simulink model "SrmAmLinearApcZhw3b1"  (R2013b)
settings: Solver=ode45  StartTime=0.0  StopTime=0.1  RelTol=1e-3
InitFcn:
  | theta0=30*2*pi/360;
  | ks=1.22;
  | is=2;
  | lu=0.016;
  | rs=1.5;
  | lux=1;
  | j=0.005;
settings Model: NumberOfSteps=5  Creator=mamingkai  LastModifiedBy=Think79

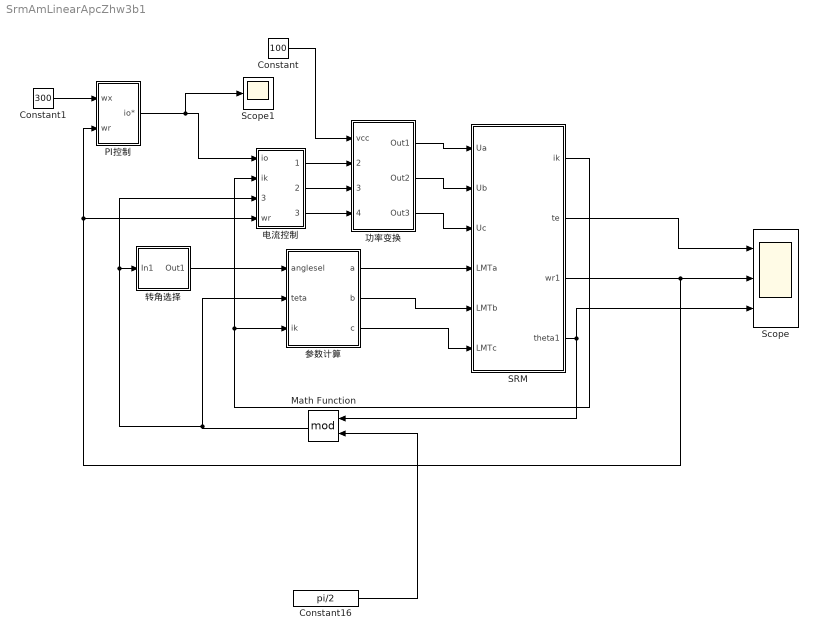
== system SrmAmLinearApcZhw3b1 ==
  Constant : Constant  Value=100
  Constant1 : Constant  Value=300
  Constant16 : Constant  Value=pi/2
  Math Function : Math  Operator=mod  SaturateOnIntegerOverflow=on
  PI控制 : Subsystem
  SRM : Subsystem
  Scope : Scope  NumInputPorts=3
      settings: YMin=-5~-5~-5  YMax=5~5~5
  Scope1 : Scope
      settings: SaveName=ScopeData3
  功率变换 : Subsystem
  参数计算 : Subsystem
  电流控制 : Subsystem
  转角选择 : Subsystem
  wires:
  Constant1/1 -> PI控制/1(wx)
  电流控制/1(Out1) -> 功率变换/2(PUSEA)
  电流控制/2(Out2) -> 功率变换/3(PUDEB)
  电流控制/3(Out3) -> 功率变换/4(PUSEC)
  PI控制/1(io*) -> Scope1/1, 电流控制/1(io)
  Constant/1 -> 功率变换/1(vcc)
  功率变换/1(Out1) -> SRM/1(Ua)
  功率变换/2(Out2) -> SRM/2(Ub)
  功率变换/3(Out3) -> SRM/3(Uc)
  转角选择/1(Out1) -> 参数计算/1("anglesel ")
  SRM/1(ik) -> 电流控制/2(ik), 参数计算/3(ik)
  SRM/3(wr1) -> PI控制/2(wr), 电流控制/4(wr), Scope/2
  Math Function/1 -> 参数计算/2(teta), 电流控制/3(teta), 转角选择/1(In1)
  SRM/2(te) -> Scope/1
  参数计算/1(a) -> SRM/4(LMTa)
  参数计算/2(b) -> SRM/5(LMTb)
  参数计算/3(c) -> SRM/6(LMTc)
  Constant16/1 -> Math Function/2
  SRM/4(theta1) -> Scope/3, Math Function/1

== system SrmAmLinearApcZhw3b1/PI控制 ==
  note: The output is the goal of Current
  wx : Inport
  wr : Inport  Port=2
  Gain : Gain
  Gain1 : Gain
  Integrator : Integrator
  Saturation : Saturate  UpperLimit=15
  netsum : Sum  Inputs=2  SaturateOnIntegerOverflow=on  InputSameDT=on  OutDataTypeStr=Inherit: Same as first input
  netsum1 : Sum  Inputs=+-  SaturateOnIntegerOverflow=on  InputSameDT=on  OutDataTypeStr=Inherit: Same as first input
  io* : Outport
  wires:
  wx/1 -> netsum1/1
  wr/1 -> netsum1/2
  netsum1/1 -> Gain/1, Gain1/1
  Gain1/1 -> Integrator/1
  Integrator/1 -> netsum/2
  Gain/1 -> netsum/1
  netsum/1 -> Saturation/1
  Saturation/1 -> io*/1

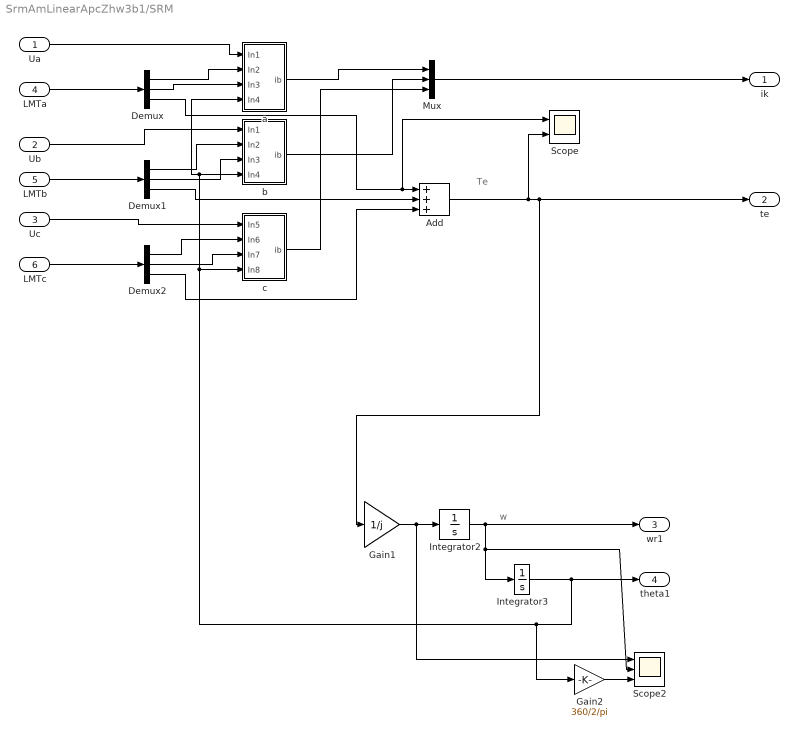
== system SrmAmLinearApcZhw3b1/SRM ==
  note: Te
  note: w
  Ua : Inport
  Ub : Inport  Port=2
  Uc : Inport  Port=3
  LMTa : Inport  Port=4
  LMTb : Inport  Port=5
  LMTc : Inport  Port=6
  Add : Sum  Inputs=+++
  Demux : Demux  Outputs=3
  Demux1 : Demux  Outputs=3
  Demux2 : Demux  Outputs=3
  Gain1 : Gain  Gain=1/j
  Gain2 : Gain  Gain=360/2/pi
  Integrator2 : Integrator
  Integrator3 : Integrator  InitialCondition=5*2*pi/360
  Mux : Mux  Inputs=3
  Scope : Scope  NumInputPorts=2
      settings: YMin=-5~-5  YMax=5~5
  Scope2 : Scope  NumInputPorts=3
      settings: YMin=-5~-5~-5  YMax=5~5~5  SaveName=ScopeData2
  a : Subsystem
  b : Subsystem
  c : Subsystem
  ik : Outport
  te : Outport  Port=2
  wr1 : Outport  Port=3
  theta1 : Outport  Port=4
  wires:
  LMTa/1 -> Demux/1
  Demux/3 -> Scope/1, Add/1
  Ub/1 -> b/1(In1)
  Demux1/1 -> b/2(In2)
  Demux1/2 -> b/3(In3)
  Demux1/3 -> Add/2
  LMTc/1 -> Demux2/1
  LMTb/1 -> Demux1/1
  Demux2/3 -> Add/3
  b/1("ib ") -> Mux/2
  Mux/1 -> ik/1
  a/1("ib ") -> Mux/1
  Demux2/2 -> c/3(In7)
  Demux2/1 -> c/2(In6)
  Uc/1 -> c/1(In5)
  c/1("ib ") -> Mux/3
  Demux/2 -> a/3(In3)
  Demux/1 -> a/2(In2)
  Ua/1 -> a/1(In1)
  Integrator2/1 -> Integrator3/1, Scope2/2, wr1/1
  Add/1 -> Gain1/1, te/1, Scope/2
  Gain1/1 -> Scope2/1, Integrator2/1
  Integrator3/1 -> a/4(In4), b/4(In4), c/4(In8), Gain2/1, theta1/1
  Gain2/1 -> Scope2/3

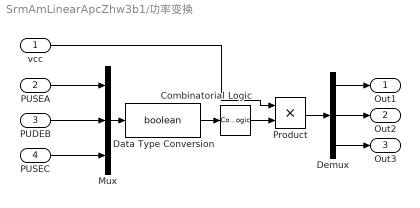
== system SrmAmLinearApcZhw3b1/功率变换 ==
  vcc : Inport
  PUSEA : Inport  Port=2
  PUDEB : Inport  Port=3
  PUSEC : Inport  Port=4
  Combinatorial Logic : CombinatorialLogic  TruthTable=[0 0 0 ;0 0 1;0 1 0;0 1 1;1 0 0;1 0 1;1 1 0;1 1 1]
  Data Type Conversion : DataTypeConversion  OutDataTypeStr=boolean
  Demux : Demux  Outputs=3
  Mux : Mux  Inputs=3
  Product : Product
  Out1 : Outport
  Out2 : Outport  Port=2
  Out3 : Outport  Port=3
  wires:
  PUSEA/1 -> Mux/1
  Demux/1 -> Out1/1
  Product/1 -> Demux/1
  Demux/2 -> Out2/1
  Demux/3 -> Out3/1
  PUDEB/1 -> Mux/2
  PUSEC/1 -> Mux/3
  Combinatorial Logic/1 -> Product/2
  vcc/1 -> Product/1
  Mux/1 -> Data Type Conversion/1
  Data Type Conversion/1 -> Combinatorial Logic/1

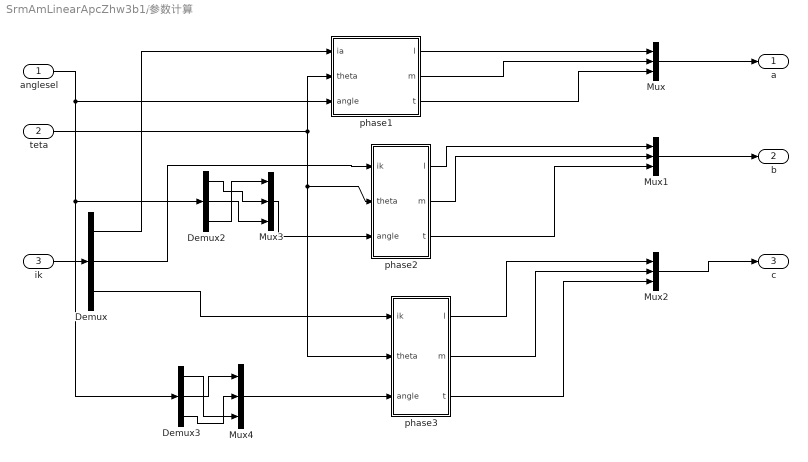
== system SrmAmLinearApcZhw3b1/参数计算 ==
  "anglesel " : Inport
  teta : Inport  Port=2
  ik : Inport  Port=3
  Demux : Demux  Outputs=3
  Demux2 : Demux  Outputs=3
  Demux3 : Demux  Outputs=3
  Mux{,1..4} (5 alike) : Mux  Inputs=3
  phase1 : Subsystem
  phase2 : Subsystem
  phase3 : Subsystem
  a : Outport
  b : Outport  Port=2
  c : Outport  Port=3
  wires:
  teta/1 -> phase3/2(theta), phase2/2(theta), phase1/2(theta)
  Mux/1 -> a/1
  ik/1 -> Demux/1
  Demux/1 -> phase1/1(ia)
  Demux/2 -> phase2/1(ik)
  Demux/3 -> phase3/1(ik)
  phase1/1(l) -> Mux/1
  phase1/2(m) -> Mux/2
  phase3/3(t) -> Mux2/3
  Mux1/1 -> b/1
  Mux2/1 -> c/1
  Demux2/1 -> Mux3/2
  Demux2/2 -> Mux3/3
  Demux2/3 -> Mux3/1
  Mux3/1 -> phase2/3(angle)
  "anglesel "/1 -> Demux2/1, Demux3/1, phase1/3(angle)
  Mux4/1 -> phase3/3(angle)
  Demux3/1 -> Mux4/3
  Demux3/2 -> Mux4/1
  Demux3/3 -> Mux4/2
  phase2/1(l) -> Mux1/1
  phase1/3(t) -> Mux/3
  phase2/2(m) -> Mux1/2
  phase2/3(t) -> Mux1/3
  phase3/1(l) -> Mux2/1
  phase3/2(m) -> Mux2/2

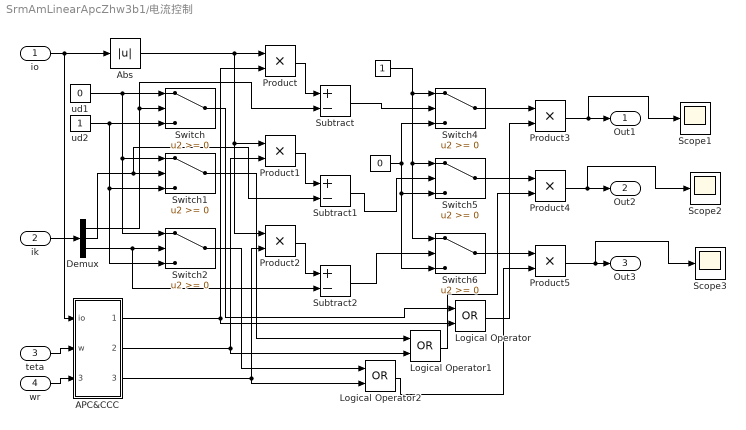
== system SrmAmLinearApcZhw3b1/电流控制 ==
  io : Inport
  ik : Inport  Port=2
  teta : Inport  Port=3
  wr : Inport  Port=4
  " " : Constant
  " " : Constant  Value=0
  APC&CCC : Subsystem
  Abs : Abs
  Demux : Demux  Outputs=3
  Logical Operator : Logic  Operator=OR  AllPortsSameDT=off  OutDataTypeStr=boolean
  Logical Operator1 : Logic  Operator=OR  AllPortsSameDT=off  OutDataTypeStr=boolean
  Logical Operator2 : Logic  Operator=OR  AllPortsSameDT=off  OutDataTypeStr=boolean
  Product{,1..5} (6 alike) : Product
  Scope1 : Scope
      settings: SaveName=ScopeData7
  Scope2 : Scope
      settings: SaveName=ScopeData8
  Scope3 : Scope
      settings: SaveName=ScopeData9
  Subtract : Sum  Inputs=+-
  Subtract1 : Sum  Inputs=+-
  Subtract2 : Sum  Inputs=+-
  Switch{,1..2,4..6} (6 alike) : Switch
  ud1 : Constant  Value=0
  ud2 : Constant
  Out1 : Outport
  Out2 : Outport  Port=2
  Out3 : Outport  Port=3
  wires:
  ik/1 -> Demux/1
  io/1 -> APC&CCC/1(io), Abs/1
  Abs/1 -> Product2/1, Product1/1, Product/1
  ud1/1 -> Switch2/1, Switch1/1, Switch/1
  ud2/1 -> Switch2/3, Switch1/3, Switch/3
  teta/1 -> APC&CCC/2(w)
  Demux/1 -> Subtract/2, Switch/2
  Demux/3 -> Subtract2/2, Switch2/2
  Demux/2 -> Subtract1/2, Switch1/2
  APC&CCC/1(Out1) -> Logical Operator/2, Product/2
  APC&CCC/2(Out2) -> Logical Operator1/2, Product1/2
  APC&CCC/3(Out3) -> Logical Operator2/2, Product2/2
  Switch/1 -> Logical Operator/1
  Switch1/1 -> Logical Operator1/1
  Switch2/1 -> Logical Operator2/1
  Product/1 -> Subtract/1
  Product1/1 -> Subtract1/1
  Product2/1 -> Subtract2/1
  " "/1 -> Switch6/1, Switch5/1, Switch4/1
  " "/1 -> Switch6/3, Switch5/3, Switch4/3
  wr/1 -> APC&CCC/3(theta)
  Logical Operator/1 -> Product3/2
  Logical Operator1/1 -> Product4/2
  Logical Operator2/1 -> Product5/2
  Switch6/1 -> Product5/1
  Switch5/1 -> Product4/1
  Switch4/1 -> Product3/1
  Product3/1 -> Scope1/1, Out1/1
  Product4/1 -> Scope2/1, Out2/1
  Product5/1 -> Scope3/1, Out3/1
  Subtract1/1 -> Switch5/2
  Subtract/1 -> Switch4/2
  Subtract2/1 -> Switch6/2

== system SrmAmLinearApcZhw3b1/转角选择 ==
  In1 : Inport
  Constant : Constant
  Constant1 : Constant  Value=0
  Mux : Mux  Inputs=3
  Mux1 : Mux  Inputs=3
  Mux2 : Mux  Inputs=3
  Switch : Switch  Threshold=pi/6
  Switch1 : Switch  Threshold=pi/3
  Switch2 : Switch  Threshold=pi/3
  Out1 : Outport
  wires:
  Constant/1 -> Mux2/3, Mux1/2, Mux/1
  Mux/1 -> Switch/3
  Constant1/1 -> Mux/3, Mux/2, Mux1/1, Mux2/2, Mux2/1, Mux1/3
  Mux1/1 -> Switch1/3, Switch/1
  Mux2/1 -> Switch1/1
  In1/1 -> Switch2/2, Switch1/2, Switch/2
  Switch/1 -> Switch2/3
  Switch1/1 -> Switch2/1
  Switch2/1 -> Out1/1

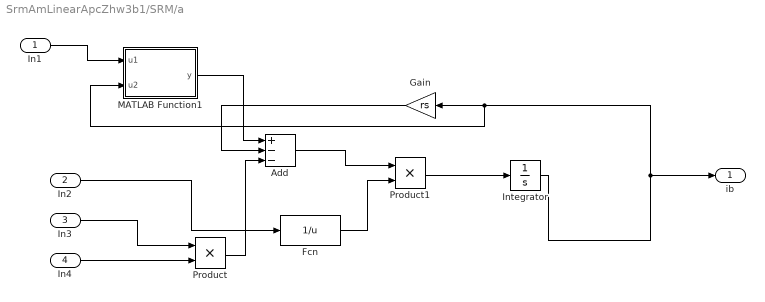
== system SrmAmLinearApcZhw3b1/SRM/a ==
  In1 : Inport
  In2 : Inport  Port=2
  In3 : Inport  Port=3
  In4 : Inport  Port=4
  Add : Sum  Inputs=+--
  Fcn : Fcn  Expr=1/u
  Gain : Gain  Gain=rs
  Integrator : Integrator  LimitOutput=on  LowerSaturationLimit=0
  MATLAB Function1 : MATLAB Function  TreatAsAtomicUnit=on
  Product : Product
  Product1 : Product
  "ib " : Outport
  wires:
  In4/1 -> Product/2
  In3/1 -> Product/1
  In2/1 -> Fcn/1
  Gain/1 -> Add/2
  Product/1 -> Add/3
  Add/1 -> Product1/1
  Fcn/1 -> Product1/2
  Integrator/1 -> MATLAB Function1/2(u2), Gain/1, "ib "/1
  MATLAB Function1/1(y) -> Add/1
  In1/1 -> MATLAB Function1/1(u1)
  Product1/1 -> Integrator/1

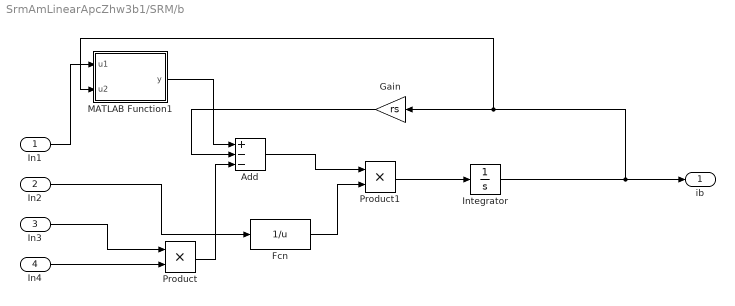
== system SrmAmLinearApcZhw3b1/SRM/b ==
  In1 : Inport
  In2 : Inport  Port=2
  In3 : Inport  Port=3
  In4 : Inport  Port=4
  Add : Sum  Inputs=+--
  Fcn : Fcn  Expr=1/u
  Gain : Gain  Gain=rs
  Integrator : Integrator  LimitOutput=on  LowerSaturationLimit=0
  MATLAB Function1 : MATLAB Function  TreatAsAtomicUnit=on
  Product : Product
  Product1 : Product
  "ib " : Outport
  wires:
  In4/1 -> Product/2
  In3/1 -> Product/1
  In2/1 -> Fcn/1
  Gain/1 -> Add/2
  Product/1 -> Add/3
  Add/1 -> Product1/1
  MATLAB Function1/1(y) -> Add/1
  In1/1 -> MATLAB Function1/1(u1)
  Fcn/1 -> Product1/2
  Product1/1 -> Integrator/1
  Integrator/1 -> MATLAB Function1/2(u2), Gain/1, "ib "/1

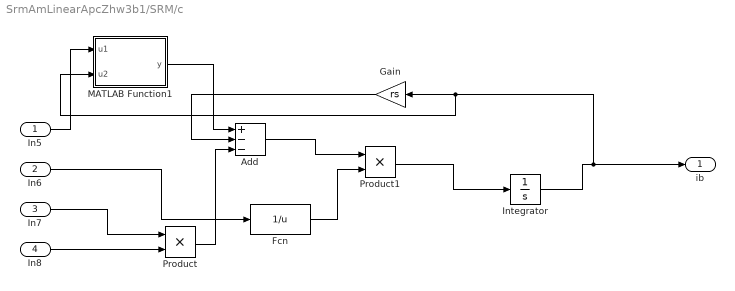
== system SrmAmLinearApcZhw3b1/SRM/c ==
  In5 : Inport
  In6 : Inport  Port=2
  In7 : Inport  Port=3
  In8 : Inport  Port=4
  Add : Sum  Inputs=+--
  Fcn : Fcn  Expr=1/u
  Gain : Gain  Gain=rs
  Integrator : Integrator  LimitOutput=on  LowerSaturationLimit=0
  MATLAB Function1 : MATLAB Function  TreatAsAtomicUnit=on
  Product : Product
  Product1 : Product
  "ib " : Outport
  wires:
  In8/1 -> Product/2
  In7/1 -> Product/1
  In6/1 -> Fcn/1
  Gain/1 -> Add/2
  Product/1 -> Add/3
  Add/1 -> Product1/1
  MATLAB Function1/1(y) -> Add/1
  In5/1 -> MATLAB Function1/1(u1)
  Fcn/1 -> Product1/2
  Integrator/1 -> MATLAB Function1/2(u2), Gain/1, "ib "/1
  Product1/1 -> Integrator/1

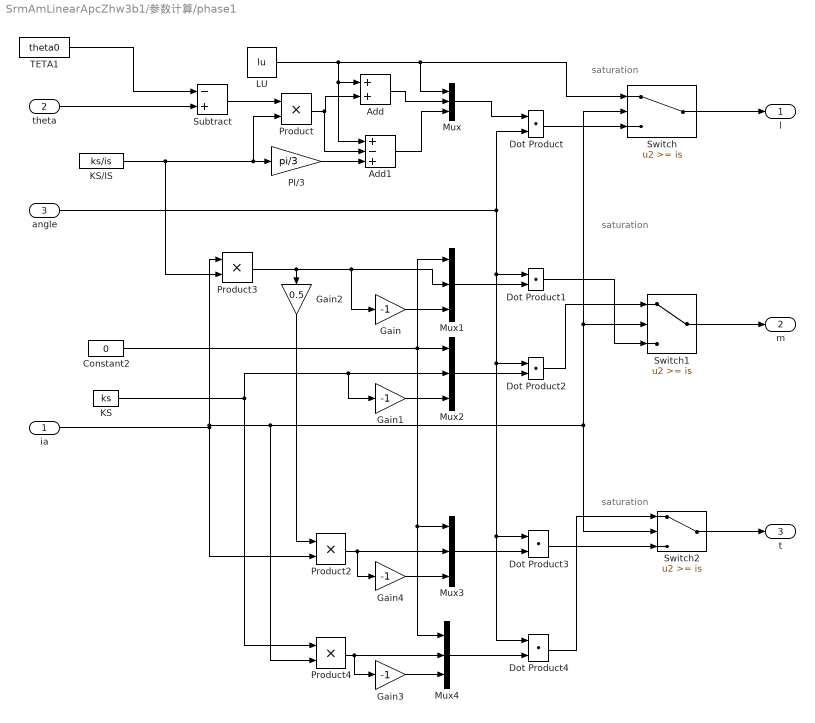
== system SrmAmLinearApcZhw3b1/参数计算/phase1 ==
  note: saturation
  note: saturation
  note: saturation
  ia : Inport
  theta : Inport  Port=2
  angle : Inport  Port=3
  Add : Sum
  Add1 : Sum  Inputs=+-+
  Constant2 : Constant  Value=0
  Dot Product{,1..4} (5 alike) : DotProduct  InputSameDT=on  OutDataTypeStr=Inherit: Inherit via internal rule
  Gain{,1,3..4} (4 alike) : Gain  Gain=-1
  Gain2 : Gain  Gain=0.5
  KS : Constant  Value=ks
  KS/IS : Constant  Value=ks/is
  LU : Constant  Value=lu
  Mux{,1..4} (5 alike) : Mux  Inputs=3
  PI/3 : Gain  Gain=pi/3
  Product{,2..4} (4 alike) : Product
  Subtract : Sum  Inputs=-+
  Switch : Switch  Threshold=is
  Switch1 : Switch  Threshold=is
  Switch2 : Switch  Threshold=is
  TETA1 : Constant  Value=theta0
  l : Outport
  m : Outport  Port=2
  t : Outport  Port=3
  wires:
  theta/1 -> Subtract/2
  TETA1/1 -> Subtract/1
  Subtract/1 -> Product/1
  KS/IS/1 -> Product3/2, PI/3/1, Product/2
  LU/1 -> Switch/1, Mux/1, Add1/1, Add/1
  Product/1 -> Add1/2, Add/2
  PI/3/1 -> Add1/3
  Add/1 -> Mux/2
  Add1/1 -> Mux/3
  Mux/1 -> Dot Product/1
  ia/1 -> Product3/1, Product4/2, Switch/2, Switch1/2, Switch2/2, Product2/2
  angle/1 -> Dot Product4/1, Dot Product3/1, Dot Product2/1, Dot Product1/1, Dot Product/2
  Mux4/1 -> Dot Product4/2
  Constant2/1 -> Mux1/1, Mux4/1, Mux3/1, Mux2/1
  Mux3/1 -> Dot Product3/2
  Mux2/1 -> Dot Product2/2
  Mux1/1 -> Dot Product1/2
  KS/1 -> Gain1/1, Mux2/2, Product4/1
  Product3/1 -> Gain/1, Mux1/2, Gain2/1
  Gain/1 -> Mux1/3
  Gain2/1 -> Product2/1
  Product4/1 -> Mux4/2, Gain3/1
  Gain3/1 -> Mux4/3
  Dot Product4/1 -> Switch2/1
  Dot Product2/1 -> Switch1/1
  Product2/1 -> Gain4/1, Mux3/2
  Gain4/1 -> Mux3/3
  Gain1/1 -> Mux2/3
  Dot Product/1 -> Switch/3
  Switch/1 -> l/1
  Dot Product1/1 -> Switch1/3
  Switch1/1 -> m/1
  Dot Product3/1 -> Switch2/3
  Switch2/1 -> t/1

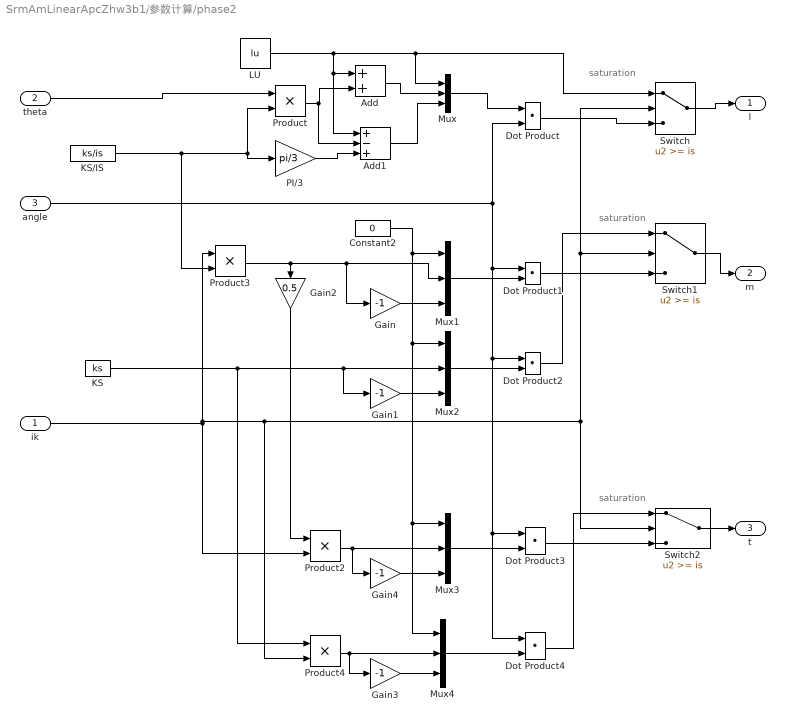
== system SrmAmLinearApcZhw3b1/参数计算/phase2 ==
  note: saturation
  note: saturation
  note: saturation
  ik : Inport
  theta : Inport  Port=2
  angle : Inport  Port=3
  Add : Sum
  Add1 : Sum  Inputs=+-+
  Constant2 : Constant  Value=0
  Dot Product{,1..4} (5 alike) : DotProduct  InputSameDT=on  OutDataTypeStr=Inherit: Inherit via internal rule
  Gain{,1,3..4} (4 alike) : Gain  Gain=-1
  Gain2 : Gain  Gain=0.5
  KS : Constant  Value=ks
  KS/IS : Constant  Value=ks/is
  LU : Constant  Value=lu
  Mux{,1..4} (5 alike) : Mux  Inputs=3
  PI/3 : Gain  Gain=pi/3
  Product{,2..4} (4 alike) : Product
  Switch : Switch  Threshold=is
  Switch1 : Switch  Threshold=is
  Switch2 : Switch  Threshold=is
  l : Outport
  m : Outport  Port=2
  t : Outport  Port=3
  wires:
  Switch/1 -> l/1
  theta/1 -> Product/1
  KS/IS/1 -> Product3/2, PI/3/1, Product/2
  LU/1 -> Switch/1, Mux/1, Add1/1, Add/1
  Product/1 -> Add1/2, Add/2
  PI/3/1 -> Add1/3
  Add/1 -> Mux/2
  Add1/1 -> Mux/3
  Mux/1 -> Dot Product/1
  Dot Product/1 -> Switch/3
  ik/1 -> Product3/1, Product4/2, Switch/2, Switch1/2, Switch2/2, Product2/2
  angle/1 -> Dot Product4/1, Dot Product3/1, Dot Product2/1, Dot Product1/1, Dot Product/2
  Mux4/1 -> Dot Product4/2
  Constant2/1 -> Mux4/1, Mux3/1, Mux2/1, Mux1/1
  Mux3/1 -> Dot Product3/2
  Mux2/1 -> Dot Product2/2
  Mux1/1 -> Dot Product1/2
  KS/1 -> Product4/1, Gain1/1, Mux2/2
  Product3/1 -> Gain/1, Mux1/2, Gain2/1
  Gain/1 -> Mux1/3
  Gain2/1 -> Product2/1
  Product4/1 -> Mux4/2, Gain3/1
  Gain3/1 -> Mux4/3
  Dot Product4/1 -> Switch2/1
  Dot Product3/1 -> Switch2/3
  Dot Product2/1 -> Switch1/1
  Dot Product1/1 -> Switch1/3
  Switch1/1 -> m/1
  Switch2/1 -> t/1
  Product2/1 -> Gain4/1, Mux3/2
  Gain4/1 -> Mux3/3
  Gain1/1 -> Mux2/3

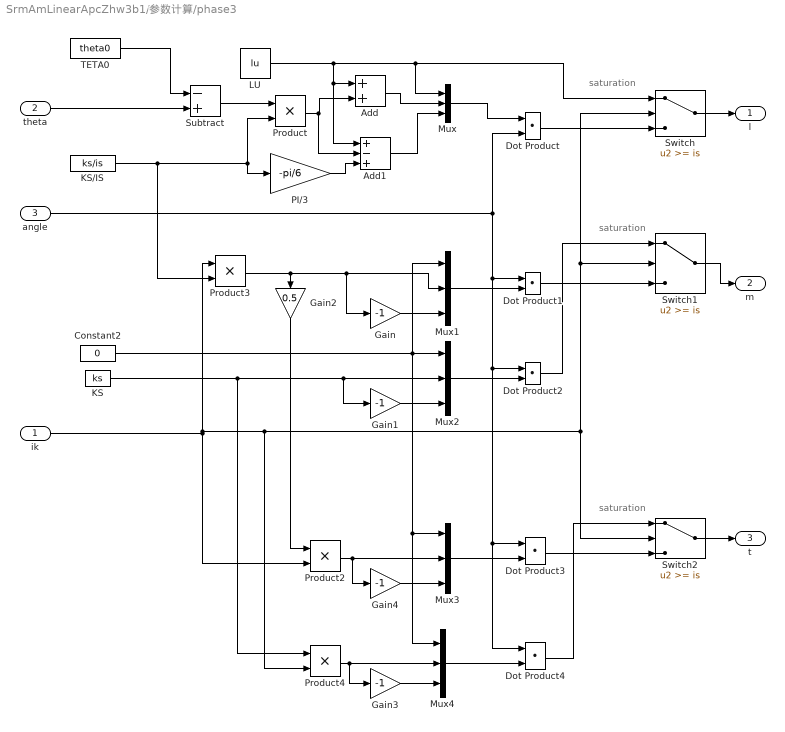
== system SrmAmLinearApcZhw3b1/参数计算/phase3 ==
  note: saturation
  note: saturation
  note: saturation
  ik : Inport
  theta : Inport  Port=2
  angle : Inport  Port=3
  Add : Sum
  Add1 : Sum  Inputs=+-+
  Constant2 : Constant  Value=0
  Dot Product{,1..4} (5 alike) : DotProduct  InputSameDT=on  OutDataTypeStr=Inherit: Inherit via internal rule
  Gain{,1,3..4} (4 alike) : Gain  Gain=-1
  Gain2 : Gain  Gain=0.5
  KS : Constant  Value=ks
  KS/IS : Constant  Value=ks/is
  LU : Constant  Value=lu
  Mux{,1..4} (5 alike) : Mux  Inputs=3
  PI/3 : Gain  Gain=-pi/6
  Product{,2..4} (4 alike) : Product
  Subtract : Sum  Inputs=-+
  Switch : Switch  Threshold=is
  Switch1 : Switch  Threshold=is
  Switch2 : Switch  Threshold=is
  TETA0 : Constant  Value=theta0
  l : Outport
  m : Outport  Port=2
  t : Outport  Port=3
  wires:
  Switch/1 -> l/1
  theta/1 -> Subtract/2
  TETA0/1 -> Subtract/1
  Subtract/1 -> Product/1
  KS/IS/1 -> Product3/2, PI/3/1, Product/2
  LU/1 -> Switch/1, Mux/1, Add1/1, Add/1
  Product/1 -> Add1/2, Add/2
  PI/3/1 -> Add1/3
  Add/1 -> Mux/2
  Add1/1 -> Mux/3
  Mux/1 -> Dot Product/1
  Dot Product/1 -> Switch/3
  ik/1 -> Product3/1, Product4/2, Switch/2, Switch1/2, Switch2/2, Product2/2
  angle/1 -> Dot Product4/1, Dot Product3/1, Dot Product2/1, Dot Product1/1, Dot Product/2
  Mux4/1 -> Dot Product4/2
  Constant2/1 -> Mux1/1, Mux4/1, Mux3/1, Mux2/1
  Mux3/1 -> Dot Product3/2
  Mux2/1 -> Dot Product2/2
  Mux1/1 -> Dot Product1/2
  KS/1 -> Product4/1, Gain1/1, Mux2/2
  Product3/1 -> Gain/1, Mux1/2, Gain2/1
  Gain/1 -> Mux1/3
  Gain2/1 -> Product2/1
  Product4/1 -> Mux4/2, Gain3/1
  Gain3/1 -> Mux4/3
  Dot Product4/1 -> Switch2/1
  Dot Product3/1 -> Switch2/3
  Dot Product2/1 -> Switch1/1
  Dot Product1/1 -> Switch1/3
  Switch1/1 -> m/1
  Switch2/1 -> t/1
  Product2/1 -> Gain4/1, Mux3/2
  Gain4/1 -> Mux3/3
  Gain1/1 -> Mux2/3

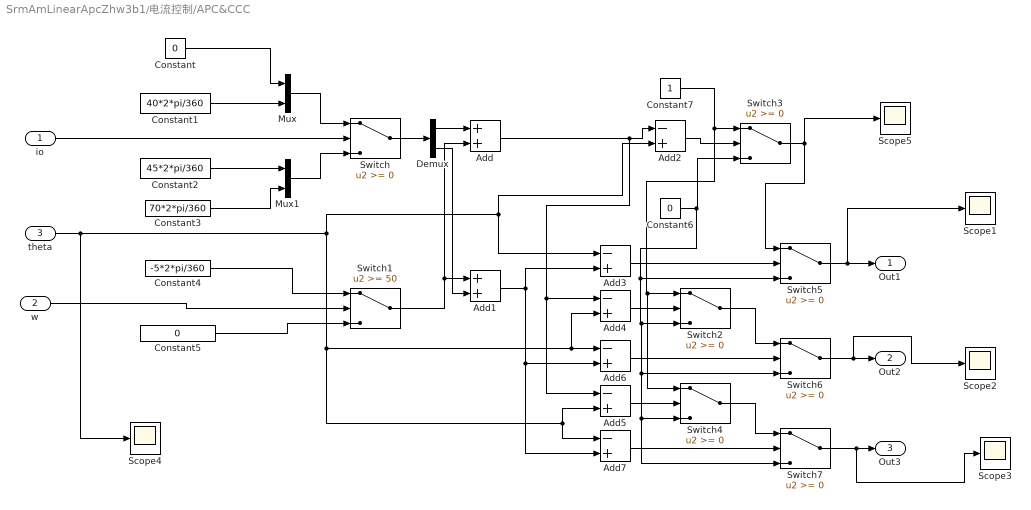
== system SrmAmLinearApcZhw3b1/电流控制/APC&CCC ==
  io : Inport
  w : Inport  Port=2
  theta : Inport  Port=3
  Add : Sum
  Add1 : Sum
  Add{2..7} (6 alike) : Sum  Inputs=-+
  Constant : Constant  Value=0
  Constant1 : Constant  Value=40*2*pi/360
  Constant2 : Constant  Value=45*2*pi/360
  Constant3 : Constant  Value=70*2*pi/360
  Constant4 : Constant  Value=-5*2*pi/360
  Constant5 : Constant  Value=0
  Constant6 : Constant  Value=0
  Constant7 : Constant
  Demux : Demux  Outputs=2
  Mux : Mux  Inputs=2
  Mux1 : Mux  Inputs=2
  Scope{1..5} (5 alike) : Scope
      Scope1 settings: SaveName=ScopeData4
      Scope2 settings: SaveName=ScopeData5
      Scope3 settings: SaveName=ScopeData6
      Scope4 settings: SaveName=ScopeData10
      Scope5 settings: SaveName=ScopeData11
  Switch{,2..7} (7 alike) : Switch
  Switch1 : Switch  Threshold=50
  Out1 : Outport
  Out2 : Outport  Port=2
  Out3 : Outport  Port=3
  wires:
  Switch5/1 -> Scope1/1, Out1/1
  w/1 -> Switch1/2
  io/1 -> Switch/2
  Mux/1 -> Switch/1
  Constant4/1 -> Switch1/1
  Constant5/1 -> Switch1/3
  Constant/1 -> Mux/1
  Constant1/1 -> Mux/2
  Constant2/1 -> Mux1/1
  Constant3/1 -> Mux1/2
  Mux1/1 -> Switch/3
  Switch/1 -> Demux/1
  Demux/1 -> Add/1
  Demux/2 -> Add1/2
  Switch1/1 -> Add1/1, Add/2
  Add1/1 -> Add3/2, Add6/2, Add7/2
  Add/1 -> Add4/1, Add5/1, Add2/1
  theta/1 -> Scope4/1, Add2/2, Add3/1, Add7/1, Add5/2, Add6/1, Add4/2
  Add3/1 -> Switch5/2
  Add4/1 -> Switch2/2
  Add6/1 -> Switch6/2
  Add5/1 -> Switch4/2
  Add7/1 -> Switch7/2
  Constant7/1 -> Switch4/1, Switch2/1, Switch3/1
  Constant6/1 -> Switch6/3, Switch7/3, Switch4/3, Switch2/3, Switch5/3, Switch3/3
  Switch2/1 -> Switch6/1
  Switch4/1 -> Switch7/1
  Switch6/1 -> Scope2/1, Out2/1
  Add2/1 -> Switch3/2
  Switch7/1 -> Scope3/1, Out3/1
  Switch3/1 -> Switch5/1, Scope5/1

== matlab function SrmAmLinearApcZhw3b1/SRM/a/MATLAB Function1 ==
  data: u1 input; y output; u2 input
function y = fcn(u1,u2)
%#codegen
if u2>0 && u1==0
    y=-100;

else
    y=u1;
end
end

== matlab function SrmAmLinearApcZhw3b1/SRM/b/MATLAB Function1 ==
  data: u1 input; y output; u2 input
function y = fcn(u1,u2)
%#codegen
if u2>0 && u1==0
    y=-100;

else
    y=u1;
end
end

== matlab function SrmAmLinearApcZhw3b1/SRM/c/MATLAB Function1 ==
  data: u1 input; y output; u2 input
function y = fcn(u1,u2)
%#codegen
if u2>0 && u1==0
    y=-100;

else
    y=u1;
end
end
